simulink model "HDD_controller_design"  (R2018b)
settings: Solver=VariableStepAuto  StartTime=0.0  StopTime=10.0  RelTol=1e-3
settings Model: Creator=luonc  LastModifiedBy=luonc

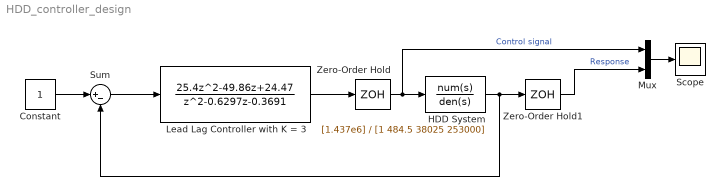
== system HDD_controller_design ==
  Constant : Constant
  HDD System : TransferFcn  Numerator=[1.437e6]  Denominator=[1 484.5 38025 253000]
  Lead Lag Controller with K = 3 : DiscreteTransferFcn  Numerator=[25.4 -49.86 24.47]  Denominator=[1 -0.6297 -0.3691]
  Mux : Mux  Inputs=2
  Scope : Scope
  Sum : Sum  Inputs=|+-
  Zero-Order Hold : ZeroOrderHold  SampleTime=0.001
  Zero-Order Hold1 : ZeroOrderHold  SampleTime=0.001
  wires:
  Zero-Order Hold/1 -> Mux/1, HDD System/1  "Control signal"
  Lead Lag Controller with K = 3/1 -> Zero-Order Hold/1
  Sum/1 -> Lead Lag Controller with K = 3/1
  HDD System/1 -> Zero-Order Hold1/1, Sum/2
  Constant/1 -> Sum/1
  Mux/1 -> Scope/1
  Zero-Order Hold1/1 -> Mux/2  "Response"
